simulink model "IdealGen_load_CtrlGen_wWT_abc_detailed_ver2"  (R2023b)
settings: Solver=VariableStepAuto  StartTime=0.0  StopTime=Tend  RelTol=1e-3
undefined symbols (not defined in the file): C_dc, c_drt, C_f, C_p_opt, f_nom, H_gen, H_vsm, H_WTR, I_dc_base, Ibase_hv, Ibase_lv, k_d_vsm, k_drt, k_p_p_vsm, k_p_q_vsm, K_pitch, Ki_cc, ki_q, Ki_vc, Kp_cc, Kp_vc, kpu, L_d, l_f, L_f, L_grid, L_mv, L_q, l_t_hvmv, l_t_mvlv, lambda_opt, Lbase1v, omega_nom, omega_WTR_min, omega_WTR_n, omega_WTR_sl, phase_shift_test_state, phase_shifts, pitch_max, pitch_min, Pitchanglevector, Pmax, Powercoefficient, psi_pm, R_a, r_f, R_grid, R_mv, r_t_hvmv, r_t_mvlv, R_WTR, rate_max, rate_min, rocof_slope, Rocof_test_state, Sbase1, Sbase_t1, T_base, T_pitch, T_servo ... (+15)
libraries: spsControlledVoltageSourceLib x6, slpidlib x6, spsPower3phInstantaneousLib x4, spsThreePhaseSeriesRLCBranchLib x4, spsThreePhaseVIMeasurementLib x3, spsRMSLib x3, spsabctodq0Lib x3, spsGroundLib x2, spsdq0toabcLib x2, spsCurrentMeasurementLib x2, spsSeriesRLCBranchLib x2, spsVoltageMeasurementLib x2
(part 2 of 2)

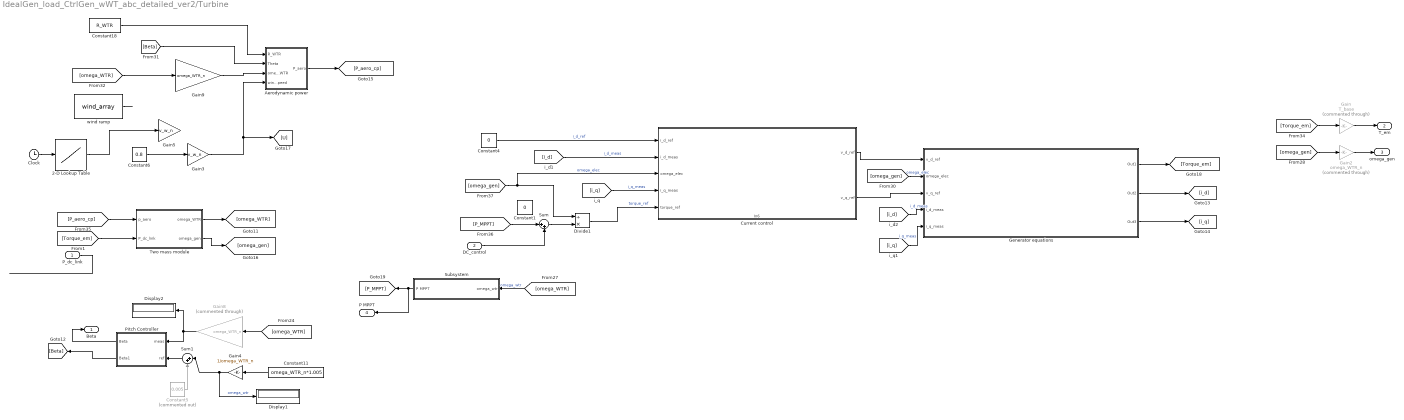
== system IdealGen_load_CtrlGen_wWT_abc_detailed_ver2/Turbine ==
  P_dc_link : Inport
  DC_control : Inport  Port=2
  2-D Lookup Table : Lookup_n-D  NumberOfTableDimensions=1  BreakpointsForDimension1=wind_array_step(1,:)  BreakpointsForDimension2=[1:3]  IndexSearchMethod=Linear search  Table=wind_array_step(2,:)  InterpMethod=Nearest  InternalRulePriority=Speed  RndMeth=Simplest
  Aerodynamic power : Subsystem
  Clock : Clock
  Constant1 : Constant  Value=0
  Constant11 : Constant  Value=omega_WTR_n*1.005
  Constant18 : Constant  Value=R_WTR
  Constant4 : Constant  Value=0
  Constant5 : Constant  Commented=on  Value=0.005
  Constant6 : Constant  Value=0.8
  Current control : Subsystem
      settings: PortSchema="{\"entries\":[{\"content\":{\"sides\":[{\"content\":{\"connectorIds\":[\"In1\",\"In2\",\"In3\",\"In4\",\"In5\"]},\"type\":\"ConnectorPlacement.EquallySpacedRectSide\",\"uuid\":\"f0c0ebaa-c967-4356-ac1b-c57f63a29779\"},{\"content\":{\"connectorIds\":[\"Out1\",\"Out2\"],\"side\":\"RIGHT\"},\"type\":\"ConnectorPlacement.EquallySpacedRectSide\",\"uuid\":\"1cdf54d9-8841-4054-96d8-98f023823611\"},{\"content\":{\"side\":\"TOP\"},\"type\":\"ConnectorPlacement.EquallySpacedRectSide\",\"uuid\":\"e5446ced-f102-4515-b1a2-d62d39d31328\"},{\"content\":{\"connectorIds\":[\"In6\"],\"side\":\"BOTTOM\"},\"type\":\"ConnectorPlacement.EquallySpacedRectSide\",\"uuid\":\"501a05db-372f-49fd-99c3-d79253c332da\"}]},\"type\":\"ConnectorPlacement.EquallySpacedConnector\",\"uuid\":\"99b5cc9b-ee78-4a5c-8cde-7a0c5c1e273f\"}],\"packageUris\":[\"http://schema.mathworks.com/mf0/Connector/R2020b\"],\"version\":\"1.0\"}"
  Display1 : Display
  Display2 : Display
  Divide1 : Product  Inputs=/*
  Gain : Gain  Commented=through  Gain=T_base
  Gain2 : Gain  Commented=through  Gain=omega_WTR_n
  Gain3 : Gain  Gain=v_w_n
  Gain4 : Gain  Gain=1/omega_WTR_n
  Gain5 : Gain  Gain=v_w_n
  Gain8 : Gain  Commented=through  Gain=omega_WTR_n
  Gain9 : Gain  Gain=omega_WTR_n
  Generator equations : Subsystem
  Pitch Controller : Subsystem
  Subsystem : Subsystem
  Sum : Sum  Inputs=|++
  Sum1 : Sum  Inputs=|++
  Two mass module : Subsystem
  wind ramp : FromWorkspace  VariableName=wind_array
  Beta : Outport
  T_em : Outport  Port=2
  omega_gen : Outport  Port=3
  P MPPT : Outport  Port=4
  wires:
  [omega_gen] -> Gain2/1
  [omega_WTR] -> Subsystem/1(omega_wtr)  "omega_wtr"
  [i_d] -> Current control/2(i_d_meas)  "i_d_meas"
  Generator equations/3(Out3) -> [i_q]
  [i_q] -> Generator equations/5(i_q_meas)  "i_q_meas"
  Pitch Controller/1(Beta) -> Beta/1
  [i_d] -> Generator equations/4(i_d_meas)  "i_d_meas"
  Constant18/1 -> Aerodynamic power/1(R_WTR)
  [omega_gen] -> Generator equations/2(omega_elec)  "omega_elec"
  Gain3/1 -> Aerodynamic power/4(wind speed), [U]
  [Torque_em] -> Two mass module/2(P_dc_link)
  Constant11/1 -> Gain4/1
  wind ramp/1 -> ?
  [P_aero_cp] -> Two mass module/1(p_aero)
  Constant4/1 -> Current control/1(i_d_ref)  "i_d_ref"
  Generator equations/1(Out1) -> [Torque_em]
  Constant5/1 -> Sum1/2
  Two mass module/1(omega_WTR) -> [omega_WTR]
  [P_MPPT] -> Sum/1
  Two mass module/2(omega_gen) -> [omega_gen]
  [omega_gen] -> Divide1/1, Current control/3(omega_elec)  "omega_elec"
  Sum1/1 -> Pitch Controller/2(ref)
  Gain4/1 -> Sum1/1, Display1/1  "omega_wtr"
  Constant6/1 -> Gain3/1
  [omega_WTR] -> Gain8/1
  Clock/1 -> 2-D Lookup Table/1
  Pitch Controller/2(Beta1) -> [Beta]
  [i_q] -> Current control/4(i_q_meas)  "i_q_meas"
  Aerodynamic power/1(P_aero) -> [P_aero_cp]
  Gain9/1 -> Aerodynamic power/3(omega_WTR)
  Gain8/1 -> Display2/1, Pitch Controller/1(meas)
  [Beta] -> Aerodynamic power/2(Theta)
  2-D Lookup Table/1 -> Gain5/1
  [Torque_em] -> Gain/1
  Subsystem/1(P MPPT) -> P MPPT/1, [P_MPPT]
  Divide1/1 -> Current control/5(torque_ref)  "torque_ref"
  Current control/1(v_d_ref) -> Generator equations/1(v_d_ref)
  Generator equations/2(Out2) -> [i_d]
  [omega_WTR] -> Gain9/1
  Current control/2(v_q_ref) -> Generator equations/3(v_q_ref)
  Gain/1 -> T_em/1
  Gain2/1 -> omega_gen/1
  Sum/1 -> Divide1/2
  P_dc_link/1 -> ?
  DC_control/1 -> Sum/2

== system IdealGen_load_CtrlGen_wWT_abc_detailed_ver2/Voltage control ==
  Qm : Inport
  Qref : Inport  Port=2
  Constant5 : Constant
  Gain8 : Gain  Gain=1/Sbase1
  Gain9 : Gain  Gain=k_p_q_vsm
  Scope : Scope  NumInputPorts=4
  Sum3 : Sum  Inputs=|-+
  Sum4 : Sum  Inputs=|++
  Transfer Fcn1 : TransferFcn  Numerator=[ki_q]  Denominator=[1 ki_q]
  Vref : Outport
  delta Q : Outport  Port=2
  wires:
  Constant5/1 -> Sum4/2
  Qm/1 -> Gain8/1
  Gain9/1 -> Scope/3, Sum4/1
  Transfer Fcn1/1 -> Scope/2, Gain9/1
  Sum3/1 -> Transfer Fcn1/1, Scope/1, delta Q/1  "delta Q"
  Sum4/1 -> Scope/4, Vref/1  "Vref"
  Qref/1 -> Sum3/2
  Gain8/1 -> Sum3/1

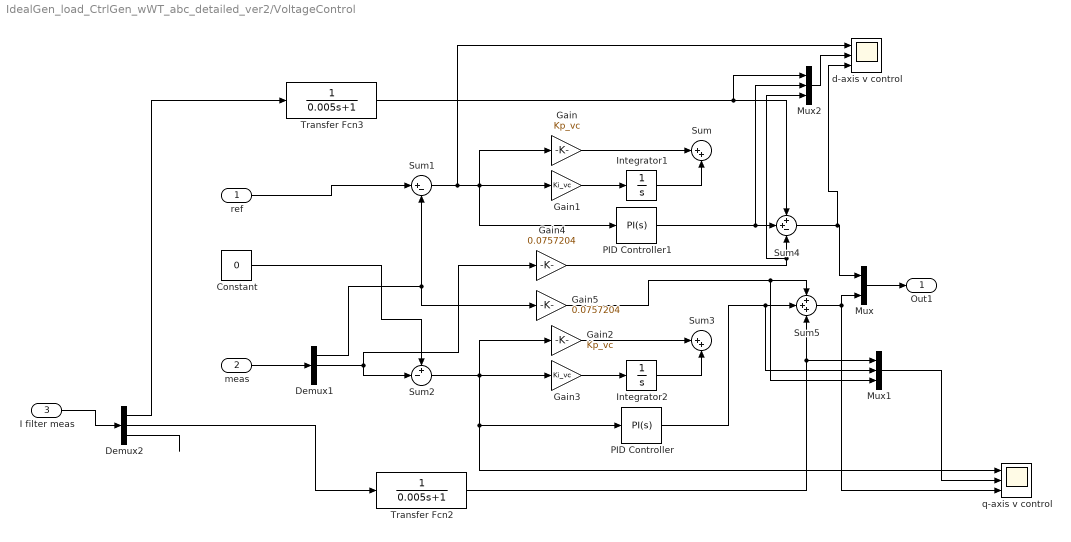
== system IdealGen_load_CtrlGen_wWT_abc_detailed_ver2/VoltageControl ==
  ref : Inport
  meas : Inport  Port=2
  I filter meas : Inport  Port=3
  Constant : Constant  Value=0
  Demux1 : Demux  Outputs=3
  Demux2 : Demux  Outputs=3
  Gain : Gain  Gain=Kp_vc
  Gain1 : Gain  Gain=Ki_vc
  Gain2 : Gain  Gain=Kp_vc
  Gain3 : Gain  Gain=Ki_vc
  Gain4 : Gain  Gain=0.0757204
  Gain5 : Gain  Gain=0.0757204
  Integrator1 : Integrator
  Integrator2 : Integrator
  Mux : Mux  Inputs=2
  Mux1 : Mux  Inputs=3
  Mux2 : Mux  Inputs=3
  PID Controller : slpidlib/PID Controller  Controller=PI  Form=Ideal  TimeDomain=Continuous-time  UseExternalTs=off  SampleTime=-1  IntegratorMethod=Forward Euler  FilterMethod=Forward Euler  ControllerParametersSource=internal  P=kpu  I=1/Tnu  UseKiTs=off  D=0  N=100  UseFilter=on  TunerSelectOption=Transfer Function Based (PID Tuner App)  InitialConditionSource=internal  InitialConditionForIntegrator=0  InitialConditionForFilter=0  DifferentiatorICPrevScaledInput=0  ExternalReset=none  TrackingMode=off  Kt=1  LimitOutput=off  SatLimitsSource=internal  UpperSaturationLimit=2  LowerSaturationLimit=-2  LinearizeAsGain=off  AntiWindupMode=none  Kb=1  LimitIntegrator=off  UpperIntegratorSaturationLimit=inf  LowerIntegratorSaturationLimit=-inf  POutMin=[]  POutMax=[]  IOutMin=[]  IOutMax=[]  DOutMin=[]  DOutMax=[]  NOutMin=[]  NOutMax=[]  SumOutMin=[]  SumOutMax=[]  SaturationOutMin=[]  SaturationOutMax=[]  PParamMin=[]  PParamMax=[]  IParamMin=[]  IParamMax=[]  DParamMin=[]  DParamMax=[]  NParamMin=[]  NParamMax=[]  KbParamMin=[]  KbParamMax=[]  KtParamMin=[]  KtParamMax=[]  KbOutMin=[]  KbOutMax=[]  KtOutMin=[]  KtOutMax=[]  IntegratorOutMin=[]  IntegratorOutMax=[]  FilterOutMin=[]  FilterOutMax=[]  SumI1OutMin=[]  SumI1OutMax=[]  SumI2OutMin=[]  SumI2OutMax=[]  SumI3OutMin=[]  SumI3OutMax=[]  SumI4OutMin=[]  SumI4OutMax=[]  SumDOutMin=[]  SumDOutMax=[]  DifferentiatorOutMin=[]  DifferentiatorOutMax=[]  FilterDiffOutCoefMin=[]  FilterDiffOutCoefMax=[]  ReciprocalOutMin=[]  ReciprocalOutMax=[]  SumDenOutMin=[]  SumDenOutMax=[]  SumNumOutMin=[]  SumNumOutMax=[]  DivideOutMin=[]  DivideOutMax=[]  UdiffTsProdOutMin=[]  UdiffTsProdOutMax=[]  NTsProdOutMin=[]  NTsProdOutMax=[]  UintegralTsProdOutMin=[]  UintegralTsProdOutMax=[]  UngainTsProdOutMin=[]  UngainTsProdOutMax=[]  ClampingZeroOutDataTypeStr=Inherit: Inherit via back propagation  ClampingZeroOutMin=[]  ClampingZeroOutMax=[]  FilterDenConstantOutDataTypeStr=Inherit: Inherit via back propagation  FilterDenConstantOutMin=[]  FilterDenConstantOutMax=[]  PCopyOutDataTypeStr=Inherit: Inherit via back propagation  PCopyOutMin=[]  PCopyOutMax=[]  NCopyOutDataTypeStr=Inherit: Inherit via back propagation  NCopyOutMin=[]  NCopyOutMax=[]  IntegratorContinuousStateAttributes=''  IntegratorStateMustResolveToSignalObject=off  IntegratorRTWStateStorageClass=Auto  FilterContinuousStateAttributes=''  FilterStateMustResolveToSignalObject=off  FilterRTWStateStorageClass=Auto  ParallelPVariant=Passthrough  IdealPVariant=InternalParameters  IVariant=InternalParameters  DVariant=Disabled  IntegratorVariant=Continuous  SatVariant=Disabled  AWVariant=Passthrough  PCopyVariant=Disabled  TRVariant=Disabled  FdbkBlocksVariant=Forward  IdealPFdbkVariant=Disabled  SatFdbkVariant=Disabled  DerivativeFilterVariant=Disabled  NVariant=Disabled  NCopyVariant=Disabled_SignalSpec  FilterICVariant=Disabled  IntegratorICVariant=InternalICs  ExternalResetVariant=Disabled  TRSumVariant=Passthrough  SumFdbkVariant=Disabled  SumVariant=Sum_PI  TsampFilterVariant=InternalTs  TsampNgainVariant=Passthrough  TsampIntegralVariant=Disabled_SignalSpec  ExternalSaturationOutDataTypeStr=Inherit: Same as second input
  PID Controller1 : slpidlib/PID Controller  Controller=PI  Form=Ideal  TimeDomain=Continuous-time  UseExternalTs=off  SampleTime=-1  IntegratorMethod=Forward Euler  FilterMethod=Forward Euler  ControllerParametersSource=internal  P=kpu  I=1/Tnu  UseKiTs=off  D=0  N=100  UseFilter=on  TunerSelectOption=Transfer Function Based (PID Tuner App)  InitialConditionSource=internal  InitialConditionForIntegrator=1  InitialConditionForFilter=0  DifferentiatorICPrevScaledInput=0  ExternalReset=none  TrackingMode=off  Kt=1  LimitOutput=off  SatLimitsSource=internal  UpperSaturationLimit=2  LowerSaturationLimit=-2  LinearizeAsGain=off  AntiWindupMode=none  Kb=1  LimitIntegrator=off  UpperIntegratorSaturationLimit=inf  LowerIntegratorSaturationLimit=-inf  POutMin=[]  POutMax=[]  IOutMin=[]  IOutMax=[]  DOutMin=[]  DOutMax=[]  NOutMin=[]  NOutMax=[]  SumOutMin=[]  SumOutMax=[]  SaturationOutMin=[]  SaturationOutMax=[]  PParamMin=[]  PParamMax=[]  IParamMin=[]  IParamMax=[]  DParamMin=[]  DParamMax=[]  NParamMin=[]  NParamMax=[]  KbParamMin=[]  KbParamMax=[]  KtParamMin=[]  KtParamMax=[]  KbOutMin=[]  KbOutMax=[]  KtOutMin=[]  KtOutMax=[]  IntegratorOutMin=[]  IntegratorOutMax=[]  FilterOutMin=[]  FilterOutMax=[]  SumI1OutMin=[]  SumI1OutMax=[]  SumI2OutMin=[]  SumI2OutMax=[]  SumI3OutMin=[]  SumI3OutMax=[]  SumI4OutMin=[]  SumI4OutMax=[]  SumDOutMin=[]  SumDOutMax=[]  DifferentiatorOutMin=[]  DifferentiatorOutMax=[]  FilterDiffOutCoefMin=[]  FilterDiffOutCoefMax=[]  ReciprocalOutMin=[]  ReciprocalOutMax=[]  SumDenOutMin=[]  SumDenOutMax=[]  SumNumOutMin=[]  SumNumOutMax=[]  DivideOutMin=[]  DivideOutMax=[]  UdiffTsProdOutMin=[]  UdiffTsProdOutMax=[]  NTsProdOutMin=[]  NTsProdOutMax=[]  UintegralTsProdOutMin=[]  UintegralTsProdOutMax=[]  UngainTsProdOutMin=[]  UngainTsProdOutMax=[]  ClampingZeroOutDataTypeStr=Inherit: Inherit via back propagation  ClampingZeroOutMin=[]  ClampingZeroOutMax=[]  FilterDenConstantOutDataTypeStr=Inherit: Inherit via back propagation  FilterDenConstantOutMin=[]  FilterDenConstantOutMax=[]  PCopyOutDataTypeStr=Inherit: Inherit via back propagation  PCopyOutMin=[]  PCopyOutMax=[]  NCopyOutDataTypeStr=Inherit: Inherit via back propagation  NCopyOutMin=[]  NCopyOutMax=[]  IntegratorContinuousStateAttributes=''  IntegratorStateMustResolveToSignalObject=off  IntegratorRTWStateStorageClass=Auto  FilterContinuousStateAttributes=''  FilterStateMustResolveToSignalObject=off  FilterRTWStateStorageClass=Auto  ParallelPVariant=Passthrough  IdealPVariant=InternalParameters  IVariant=InternalParameters  DVariant=Disabled  IntegratorVariant=Continuous  SatVariant=Disabled  AWVariant=Passthrough  PCopyVariant=Disabled  TRVariant=Disabled  FdbkBlocksVariant=Forward  IdealPFdbkVariant=Disabled  SatFdbkVariant=Disabled  DerivativeFilterVariant=Disabled  NVariant=Disabled  NCopyVariant=Disabled_SignalSpec  FilterICVariant=Disabled  IntegratorICVariant=InternalICs  ExternalResetVariant=Disabled  TRSumVariant=Passthrough  SumFdbkVariant=Disabled  SumVariant=Sum_PI  TsampFilterVariant=InternalTs  TsampNgainVariant=Passthrough  TsampIntegralVariant=Disabled_SignalSpec  ExternalSaturationOutDataTypeStr=Inherit: Same as second input
  Sum : Sum  Inputs=|++
  Sum1 : Sum  Inputs=|+-
  Sum2 : Sum  Inputs=+-|
  Sum3 : Sum  Inputs=|++
  Sum4 : Sum  Inputs=++-
  Sum5 : Sum  Inputs=+++
  Transfer Fcn2 : TransferFcn  Denominator=[0.005 1]
  Transfer Fcn3 : TransferFcn  Denominator=[0.005 1]
  d-axis v control : Scope  NumInputPorts=3
  q-axis v control : Scope  NumInputPorts=3
  Out1 : Outport
  wires:
  Demux2/1 -> Transfer Fcn3/1
  I filter meas/1 -> Demux2/1
  Sum5/1 -> Mux/2, q-axis v control/3
  Demux2/2 -> Transfer Fcn2/1
  Sum4/1 -> Mux/1, d-axis v control/3
  Sum2/1 -> PID Controller/1, q-axis v control/1, Gain3/1, Gain2/1
  Gain2/1 -> Sum3/1
  Integrator2/1 -> Sum3/2
  Gain3/1 -> Integrator2/1
  PID Controller/1 -> Mux1/2, Sum5/2
  ref/1 -> Sum1/1
  Constant/1 -> Sum2/1
  Demux1/2 -> Sum2/2, Gain4/1
  meas/1 -> Demux1/1
  Sum1/1 -> PID Controller1/1, Gain/1, Gain1/1, d-axis v control/1
  Gain1/1 -> Integrator1/1
  Integrator1/1 -> Sum/2
  Gain/1 -> Sum/1
  Mux/1 -> Out1/1
  Demux2/3 -> ?
  Gain4/1 -> Mux2/3, Sum4/3
  Gain5/1 -> Mux1/3, Sum5/1
  Demux1/1 -> Sum1/2, Gain5/1
  PID Controller1/1 -> Mux2/2, Sum4/2
  Transfer Fcn3/1 -> Mux2/1, Sum4/1
  Mux1/1 -> q-axis v control/2
  Mux2/1 -> d-axis v control/2
  Transfer Fcn2/1 -> Sum5/3, Mux1/1

== system IdealGen_load_CtrlGen_wWT_abc_detailed_ver2/WT power ==
  I_dc : Inport
  Controlled Current Source : spsControlledCurrentSourceLib/Controlled Current Source  Initialize=on  Source_Type=DC  Amplitude=0  Phase=0  Frequency=0  Measurements=None
  Current Measurement1 : spsCurrentMeasurementLib/Current Measurement  PhasorSimulation=off  OutputType=Complex  PSBequivalent=0
  Memory1 : Memory  InitialCondition=V_dc
  Product1 : Product  SaturateOnIntegerOverflow=on  OutDataTypeStr=Inherit: Same as first input
  Voltage Measurement1 : spsVoltageMeasurementLib/Voltage Measurement  PhasorSimulation=off  OutputType=Complex  PSBequivalent=0
  + : PMIOPort  Side=Right
  - : PMIOPort  Port=2  Side=Right
  Pwt : Outport
  V_dc : Outport  Port=2
  i_dc_meas : Outport  Port=3
  wires:
  Current Measurement1/1 -> i_dc_meas/1, Product1/1
  Product1/1 -> Pwt/1
  Voltage Measurement1/1 -> Memory1/1, Product1/2
  I_dc/1 -> Controlled Current Source/1
  Memory1/1 -> V_dc/1
  connections:
  Controlled Current Source/LConn1 -- Voltage Measurement1/LConn2 -- -/RConn1
  Voltage Measurement1/LConn1 -- Current Measurement1/RConn1 -- +/RConn1
  Controlled Current Source/RConn1 -- Current Measurement1/LConn1

== system IdealGen_load_CtrlGen_wWT_abc_detailed_ver2/constant DC Voltage ==
  DC Voltage Source2 : spsDCVoltageSourceLib/DC Voltage Source  Amplitude=V_dc/2  Measurements=None
  DC Voltage Source3 : spsDCVoltageSourceLib/DC Voltage Source  Amplitude=V_dc/2  Measurements=None
  + : PMIOPort  Side=Left
  - : PMIOPort  Port=2  Side=Right
  connections:
  DC Voltage Source2/LConn1 -- DC Voltage Source3/RConn1
  DC Voltage Source2/RConn1 -- +/RConn1
  DC Voltage Source3/LConn1 -- -/RConn1

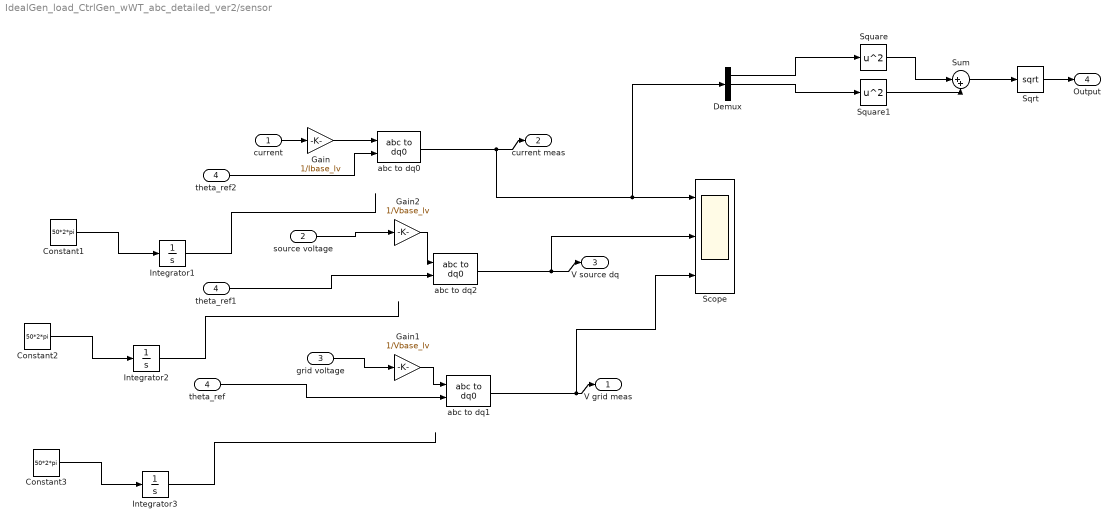
== system IdealGen_load_CtrlGen_wWT_abc_detailed_ver2/sensor ==
  current : Inport
  source voltage : Inport  Port=2
  grid voltage : Inport  Port=3
  theta_ref : Inport  Port=4
  Constant1 : Constant  Value=50*2*pi
  Constant2 : Constant  Value=50*2*pi
  Constant3 : Constant  Value=50*2*pi
  Demux : Demux  Outputs=3
  Gain : Gain  Gain=1/Ibase_lv
  Gain1 : Gain  Gain=1/Vbase_lv
  Gain2 : Gain  Gain=1/Vbase_lv
  Integrator1 : Integrator
  Integrator2 : Integrator
  Integrator3 : Integrator
  Scope : Scope  NumInputPorts=3
  Sqrt : Sqrt
  Square : Math  Operator=square
  Square1 : Math  Operator=square
  Sum : Sum  Inputs=|++
  abc to dq0 : spsabctodq0Lib/abc to dq0  Alignment=90 degrees behind phase A axis
  abc to dq1 : spsabctodq0Lib/abc to dq0  Alignment=90 degrees behind phase A axis
  abc to dq2 : spsabctodq0Lib/abc to dq0  Alignment=90 degrees behind phase A axis
  theta_ref1 : InportShadow  Port=4
  theta_ref2 : InportShadow  Port=4
  V grid meas : Outport
  current meas : Outport  Port=2
  V source dq : Outport  Port=3
  Output : Outport  Port=4
  wires:
  Gain/1 -> abc to dq0/1
  abc to dq0/1 -> Demux/1, Scope/1, current meas/1
  abc to dq1/1 -> Scope/3, V grid meas/1
  grid voltage/1 -> Gain1/1
  source voltage/1 -> Gain2/1
  abc to dq2/1 -> Scope/2, V source dq/1
  Integrator1/1 -> ?
  Constant1/1 -> Integrator1/1
  theta_ref/1 -> abc to dq1/2
  theta_ref1/1 -> abc to dq2/2
  theta_ref2/1 -> abc to dq0/2
  Constant2/1 -> Integrator2/1
  Integrator2/1 -> ?
  Integrator3/1 -> ?
  Constant3/1 -> Integrator3/1
  Gain2/1 -> abc to dq2/1
  current/1 -> Gain/1
  Gain1/1 -> abc to dq1/1
  Demux/1 -> Square/1
  Demux/2 -> Square1/1
  Square/1 -> Sum/1
  Square1/1 -> Sum/2
  Sum/1 -> Sqrt/1
  Sqrt/1 -> Output/1

== system IdealGen_load_CtrlGen_wWT_abc_detailed_ver2/DC-link voltage controller/DC init ==
  second : Inport
  init : Inport  Port=2
  Clock : Clock
  Switch : Switch  Criteria=u2 > Threshold  Threshold=10  SaturateOnIntegerOverflow=off  InputSameDT=off
  "   " : Outport
  wires:
  second/1 -> Switch/1
  init/1 -> Switch/3
  Clock/1 -> Switch/2
  Switch/1 -> "   "/1

== system IdealGen_load_CtrlGen_wWT_abc_detailed_ver2/Turbine/Aerodynamic power ==
  note: P = 0.5*rho*A*cp(lambda,beta)*U^3
  R_WTR : Inport
  Theta : Inport  Port=2
  omega_WTR : Inport  Port=3
  wind speed : Inport  Port=4
  2-D Lookup Table1 : Lookup_n-D  BreakpointsForDimension1=TSRvector  BreakpointsForDimension2=Pitchanglevector  Table=Powercoefficient  InternalRulePriority=Speed  RndMeth=Simplest
      settings: InputPortMap=u0,u1
  CP_calculator : MATLAB Function  TreatAsAtomicUnit=on
  CP_live : Scope  NumInputPorts=4
  Gain5 : Gain  Gain=1/v_w_n
  Gain7 : Gain  Gain=1/15e6
  MATLAB Function2 : MATLAB Function  TreatAsAtomicUnit=on
  Mux : Mux  Inputs=2
  P_aero_scope : Scope  NumInputPorts=3
  lambda_cal : MATLAB Function  TreatAsAtomicUnit=on
  P_aero : Outport
  wires:
  R_WTR/1 -> CP_calculator/2(R_WTR), MATLAB Function2/1(R_WTR)
  wind speed/1 -> Gain5/1, MATLAB Function2/3(U), CP_calculator/4(U), CP_live/3
  Theta/1 -> 2-D Lookup Table1/2, CP_live/1, CP_calculator/1(Theta)
  omega_WTR/1 -> CP_calculator/3(omega_WTR), CP_live/2
  MATLAB Function2/1(P_aero) -> Gain7/1
  CP_calculator/2(lambda) -> CP_live/4, 2-D Lookup Table1/1
  Gain7/1 -> P_aero_scope/1, P_aero/1  "p_aero [pu]"
  CP_calculator/1(cp) -> Mux/1
  Gain5/1 -> P_aero_scope/2  "Wind speed [pu]"
  2-D Lookup Table1/1 -> Mux/2, MATLAB Function2/2(cp)
  Mux/1 -> P_aero_scope/3  "Cp [pu]"

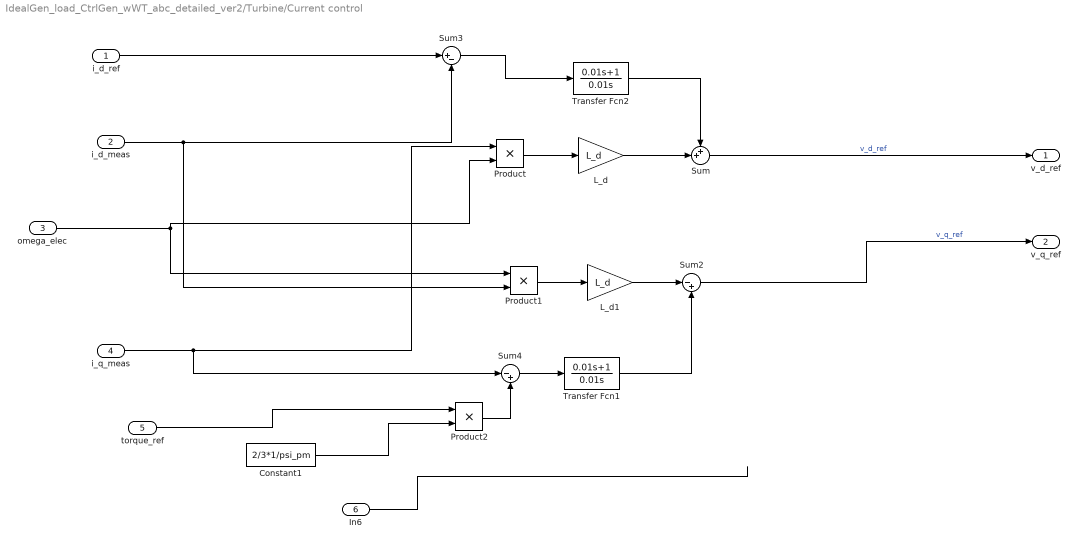
== system IdealGen_load_CtrlGen_wWT_abc_detailed_ver2/Turbine/Current control ==
  i_d_ref : Inport
  i_d_meas : Inport  Port=2
  omega_elec : Inport  Port=3
  i_q_meas : Inport  Port=4
  torque_ref : Inport  Port=5
  In6 : Inport  Port=6
  Constant1 : Constant  Value=2/3*1/psi_pm
  L_d : Gain  Gain=L_d
  L_d1 : Gain  Gain=L_d
  Product : Product
  Product1 : Product
  Product2 : Product
  Sum : Sum  Inputs=++|
  Sum2 : Sum  Inputs=|-+
  Sum3 : Sum  Inputs=|+-
  Sum4 : Sum  Inputs=|-+
  Transfer Fcn1 : TransferFcn  Numerator=[0.01 1]  Denominator=[0.01 0]
  Transfer Fcn2 : TransferFcn  Numerator=[0.01 1]  Denominator=[0.01 0]
  v_d_ref : Outport
  v_q_ref : Outport  Port=2
  wires:
  Sum3/1 -> Transfer Fcn2/1
  L_d1/1 -> Sum2/1
  Transfer Fcn2/1 -> Sum/1
  omega_elec/1 -> Product/2, Product1/1
  Constant1/1 -> Product2/2
  Sum4/1 -> Transfer Fcn1/1
  Product2/1 -> Sum4/2
  Product/1 -> L_d/1
  Sum/1 -> v_d_ref/1  "v_d_ref"
  Transfer Fcn1/1 -> Sum2/2
  i_d_meas/1 -> Product1/2, Sum3/2
  Product1/1 -> L_d1/1
  L_d/1 -> Sum/2
  i_q_meas/1 -> Sum4/1, Product/1
  i_d_ref/1 -> Sum3/1
  torque_ref/1 -> Product2/1
  Sum2/1 -> v_q_ref/1  "v_q_ref"
  In6/1 -> ?

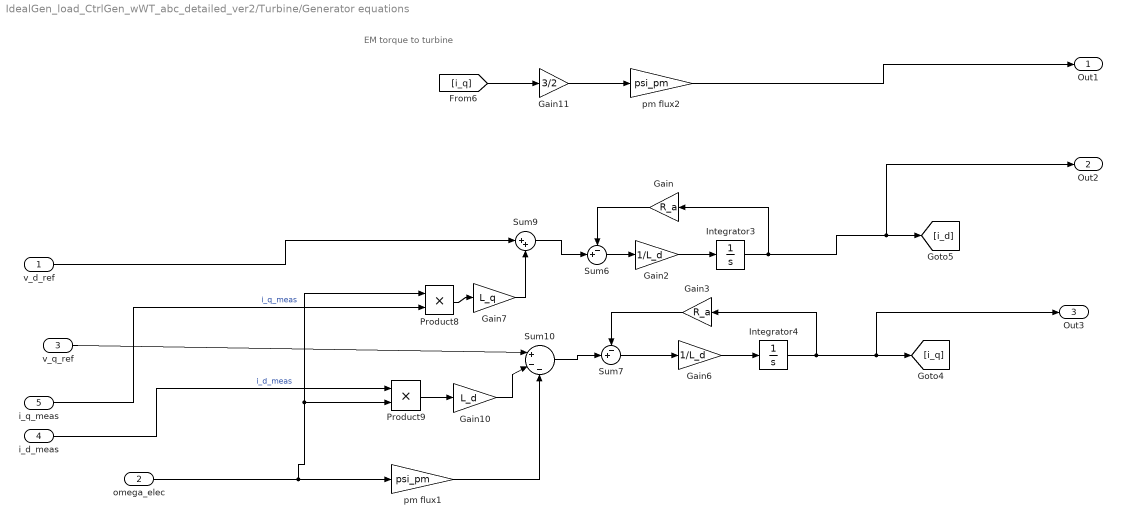
== system IdealGen_load_CtrlGen_wWT_abc_detailed_ver2/Turbine/Generator equations ==
  note: EM torque to turbine
  v_d_ref : Inport
  omega_elec : Inport  Port=2
  v_q_ref : Inport  Port=3
  i_d_meas : Inport  Port=4
  i_q_meas : Inport  Port=5
  Gain : Gain  Gain=R_a
  Gain10 : Gain  Gain=L_d
  Gain11 : Gain  Gain=3/2
  Gain2 : Gain  Gain=1/L_d
  Gain3 : Gain  Gain=R_a
  Gain6 : Gain  Gain=1/L_d
  Gain7 : Gain  Gain=L_q
  Integrator3 : Integrator
  Integrator4 : Integrator  InitialCondition=2.3e4
  Product8 : Product
  Product9 : Product
  Sum10 : Sum  Inputs=|+--
  Sum6 : Sum  Inputs=-+|
  Sum7 : Sum  Inputs=-+|
  Sum9 : Sum  Inputs=|++
  pm flux1 : Gain  Gain=psi_pm
  pm flux2 : Gain  Gain=psi_pm
  Out1 : Outport
  Out2 : Outport  Port=2
  Out3 : Outport  Port=3
  wires:
  Gain6/1 -> Integrator4/1
  Integrator4/1 -> Out3/1, [i_q], Gain3/1
  Sum10/1 -> Sum7/2
  v_d_ref/1 -> Sum9/1
  Product8/1 -> Gain7/1
  Sum7/1 -> Gain6/1
  Gain2/1 -> Integrator3/1
  pm flux1/1 -> Sum10/3
  Sum9/1 -> Sum6/2
  omega_elec/1 -> Product8/1, Product9/2, pm flux1/1
  [i_q] -> Gain11/1
  Gain3/1 -> Sum7/1
  Gain11/1 -> pm flux2/1
  Sum6/1 -> Gain2/1
  Gain10/1 -> Sum10/2
  Gain/1 -> Sum6/1
  Integrator3/1 -> Gain/1, Out2/1, [i_d]
  Product9/1 -> Gain10/1
  i_q_meas/1 -> Product8/2  "i_q_meas"
  i_d_meas/1 -> Product9/1  "i_d_meas"
  Gain7/1 -> Sum9/2
  v_q_ref/1 -> Sum10/1
  pm flux2/1 -> Out1/1

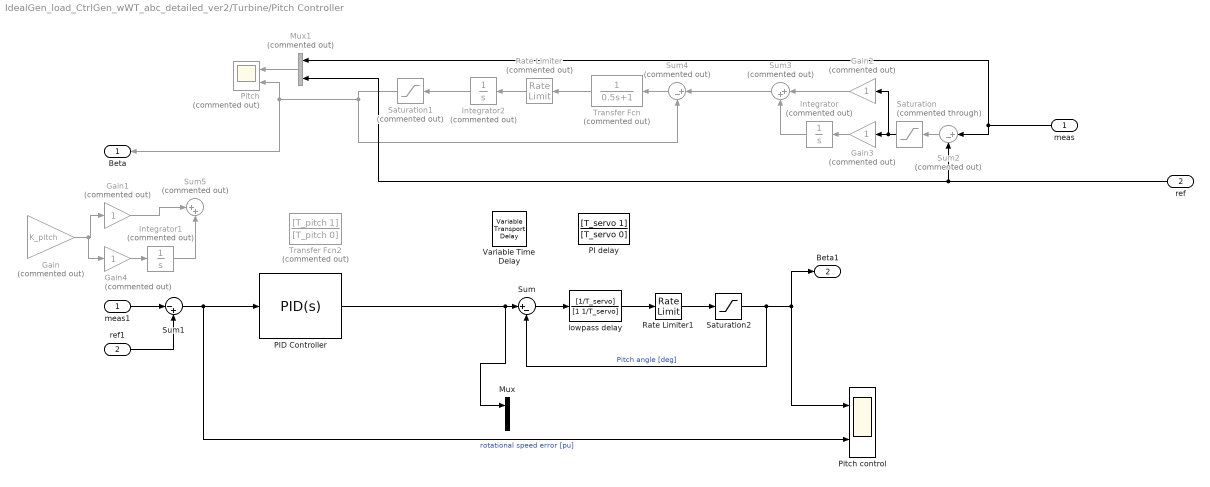
== system IdealGen_load_CtrlGen_wWT_abc_detailed_ver2/Turbine/Pitch Controller ==
  meas : Inport
  ref : Inport  Port=2
  Gain : Gain  Commented=on  Gain=K_pitch
  Gain{1..4} (4 alike) : Gain  Commented=on
  Integrator : Integrator  Commented=on
  Integrator1 : Integrator  Commented=on  LimitOutput=on  UpperSaturationLimit=pitch_max  LowerSaturationLimit=pitch_min
  Integrator2 : Integrator  Commented=on
  Mux : Mux  Inputs=2
  Mux1 : Mux  Commented=on  Inputs=2
  PI delay : TransferFcn  Numerator=[T_servo 1]  Denominator=[T_servo 0]
  PID Controller : slpidlib/PID Controller  Controller=PID  Form=Ideal  TimeDomain=Continuous-time  UseExternalTs=off  SampleTime=-1  IntegratorMethod=Forward Euler  FilterMethod=Forward Euler  ControllerParametersSource=internal  P=K_pitch  I=T_pitch  UseKiTs=on  D=0  N=100  UseFilter=on  TunerSelectOption=Transfer Function Based (PID Tuner App)  InitialConditionSource=internal  InitialConditionForIntegrator=0  InitialConditionForFilter=0  DifferentiatorICPrevScaledInput=0  ExternalReset=none  TrackingMode=off  Kt=1  LimitOutput=on  SatLimitsSource=internal  UpperSaturationLimit=pitch_max  LowerSaturationLimit=pitch_min  LinearizeAsGain=on  AntiWindupMode=clamping  Kb=1  LimitIntegrator=off  UpperIntegratorSaturationLimit=inf  LowerIntegratorSaturationLimit=-inf  POutMin=[]  POutMax=[]  IOutMin=[]  IOutMax=[]  DOutMin=[]  DOutMax=[]  NOutMin=[]  NOutMax=[]  SumOutMin=[]  SumOutMax=[]  SaturationOutMin=[]  SaturationOutMax=[]  PParamMin=[]  PParamMax=[]  IParamMin=[]  IParamMax=[]  DParamMin=[]  DParamMax=[]  NParamMin=[]  NParamMax=[]  KbParamMin=[]  KbParamMax=[]  KtParamMin=[]  KtParamMax=[]  KbOutMin=[]  KbOutMax=[]  KtOutMin=[]  KtOutMax=[]  IntegratorOutMin=[]  IntegratorOutMax=[]  FilterOutMin=[]  FilterOutMax=[]  SumI1OutMin=[]  SumI1OutMax=[]  SumI2OutMin=[]  SumI2OutMax=[]  SumI3OutMin=[]  SumI3OutMax=[]  SumI4OutMin=[]  SumI4OutMax=[]  SumDOutMin=[]  SumDOutMax=[]  DifferentiatorOutMin=[]  DifferentiatorOutMax=[]  FilterDiffOutCoefMin=[]  FilterDiffOutCoefMax=[]  ReciprocalOutMin=[]  ReciprocalOutMax=[]  SumDenOutMin=[]  SumDenOutMax=[]  SumNumOutMin=[]  SumNumOutMax=[]  DivideOutMin=[]  DivideOutMax=[]  UdiffTsProdOutMin=[]  UdiffTsProdOutMax=[]  NTsProdOutMin=[]  NTsProdOutMax=[]  UintegralTsProdOutMin=[]  UintegralTsProdOutMax=[]  UngainTsProdOutMin=[]  UngainTsProdOutMax=[]  ClampingZeroOutDataTypeStr=Inherit: Inherit via back propagation  ClampingZeroOutMin=[]  ClampingZeroOutMax=[]  FilterDenConstantOutDataTypeStr=Inherit: Inherit via back propagation  FilterDenConstantOutMin=[]  FilterDenConstantOutMax=[]  PCopyOutDataTypeStr=Inherit: Inherit via back propagation  PCopyOutMin=[]  PCopyOutMax=[]  NCopyOutDataTypeStr=Inherit: Inherit via back propagation  NCopyOutMin=[]  NCopyOutMax=[]  IntegratorContinuousStateAttributes=''  IntegratorStateMustResolveToSignalObject=off  IntegratorRTWStateStorageClass=Auto  FilterContinuousStateAttributes=''  FilterStateMustResolveToSignalObject=off  FilterRTWStateStorageClass=Auto  ParallelPVariant=Passthrough  IdealPVariant=InternalParameters  IVariant=InternalParameters  DVariant=InternalParameters  IntegratorVariant=Continuous  SatVariant=Enabled  AWVariant=ContClampingIdeal  PCopyVariant=InternalParamsIdeal  TRVariant=Disabled  FdbkBlocksVariant=Forward  IdealPFdbkVariant=Disabled  SatFdbkVariant=Disabled  DerivativeFilterVariant=ContFilter  NVariant=InternalParameters  NCopyVariant=Disabled  FilterICVariant=InternalICsFilter  IntegratorICVariant=InternalICs  ExternalResetVariant=Disabled  TRSumVariant=Passthrough  SumFdbkVariant=Disabled  SumVariant=Sum_PID  TsampFilterVariant=InternalTs  TsampNgainVariant=Passthrough  TsampIntegralVariant=Disabled_SignalSpec  ExternalSaturationOutDataTypeStr=Inherit: Same as second input
  Pitch : Scope  Commented=on  NumInputPorts=2
  Pitch control : Scope  NumInputPorts=2
  Rate Limiter : RateLimiter  Commented=on  RisingSlewLimit=5  FallingSlewLimit=-5  SampleTimeMode=inherited
  Rate Limiter1 : RateLimiter  RisingSlewLimit=rate_max  FallingSlewLimit=rate_min  SampleTimeMode=inherited
  Saturation : Saturate  Commented=through  UpperLimit=inf  LowerLimit=0
  Saturation1 : Saturate  Commented=on  UpperLimit=90  LowerLimit=0
  Saturation2 : Saturate  UpperLimit=pitch_max  LowerLimit=pitch_min
  Sum : Sum  Inputs=|+-
  Sum1 : Sum  Inputs=|-+
  Sum2 : Sum  Commented=on  Inputs=|+-
  Sum3 : Sum  Commented=on  Inputs=|++
  Sum4 : Sum  Commented=on  Inputs=|+-
  Sum5 : Sum  Commented=on  Inputs=|++
  Transfer Fcn : TransferFcn  Commented=on  Denominator=[0.5 1]
  Transfer Fcn2 : TransferFcn  Commented=on  Numerator=[T_pitch 1]  Denominator=[T_pitch 0]
  Variable Time Delay : VariableTransportDelay  MaximumDelay=T_servo
  lowpass delay : TransferFcn  Numerator=[1/T_servo]  Denominator=[1 1/T_servo]
  meas1 : InportShadow
  ref1 : InportShadow  Port=2
  Beta : Outport
  Beta1 : Outport  Port=2
  wires:
  Transfer Fcn/1 -> Rate Limiter/1
  meas/1 -> Sum2/1, Mux1/1
  Mux1/1 -> Pitch/1
  Sum2/1 -> Saturation/1
  Sum3/1 -> Sum4/1
  Saturation/1 -> Gain2/1, Gain3/1
  Saturation1/1 -> Beta/1, Pitch/2, Sum4/2
  Gain3/1 -> Integrator/1
  Gain2/1 -> Sum3/1
  Sum4/1 -> Transfer Fcn/1
  Rate Limiter/1 -> Integrator2/1
  Integrator/1 -> Sum3/2
  ref/1 -> Mux1/2, Sum2/2
  Integrator2/1 -> Saturation1/1
  Rate Limiter1/1 -> Saturation2/1
  Sum/1 -> lowpass delay/1
  lowpass delay/1 -> Rate Limiter1/1
  Saturation2/1 -> Beta1/1, Pitch control/1, Sum/2  "Pitch angle [deg]"
  meas1/1 -> Sum1/1
  ref1/1 -> Sum1/2
  PID Controller/1 -> Mux/1, Sum/1
  Sum1/1 -> PID Controller/1, Pitch control/2  "rotational speed error [pu]"
  Gain4/1 -> Integrator1/1
  Gain1/1 -> Sum5/1
  Integrator1/1 -> Sum5/2
  Gain/1 -> Gain4/1, Gain1/1

== system IdealGen_load_CtrlGen_wWT_abc_detailed_ver2/Turbine/Subsystem ==
  omega_wtr : Inport
  Constant12 : Constant  Value=R_WTR
  Constant13 : Constant  Value=lambda_opt
  Constant14 : Constant  Value=omega_WTR_n
  Constant15 : Constant  Value=omega_WTR_min
  Constant16 : Constant  Value=omega_WTR_sl
  Constant17 : Constant  Value=C_p_opt
  Gain10 : Gain  Commented=through  Gain=omega_WTR_n
  Gain11 : Gain  Commented=through  Gain=1/omega_WTR_n
  Gain12 : Gain  Gain=omega_WTR_n
  Gain6 : Gain  Gain=1/omega_WTR_n
  Gain7 : Gain  Gain=1/15e6
  MATLAB Function1 : MATLAB Function  TreatAsAtomicUnit=on
  MPPT : Scope  NumInputPorts=4
  P MPPT : Outport
  wires:
  Constant17/1 -> MATLAB Function1/6(cp_max)
  MATLAB Function1/2(b) -> MPPT/3
  Constant13/1 -> MATLAB Function1/4(lambda_opt)
  Gain6/1 -> MPPT/2  "omega_wtr"
  Gain7/1 -> P MPPT/1, MPPT/1
  Gain12/1 -> MATLAB Function1/7(omega_WTR), Gain6/1  "omega_wtr"
  Gain11/1 -> MATLAB Function1/3(omega_WTR_sl)  "omega_wtr"
  MATLAB Function1/1(P_MPPT) -> Gain7/1
  Constant15/1 -> MATLAB Function1/1(omega_WTR_min)
  Gain10/1 -> MATLAB Function1/2(omega_WTR_n)  "omega_wtr"
  Constant14/1 -> Gain10/1
  Constant16/1 -> Gain11/1
  Constant12/1 -> MATLAB Function1/5(R_WTR)
  MATLAB Function1/3(slope) -> MPPT/4
  omega_wtr/1 -> Gain12/1

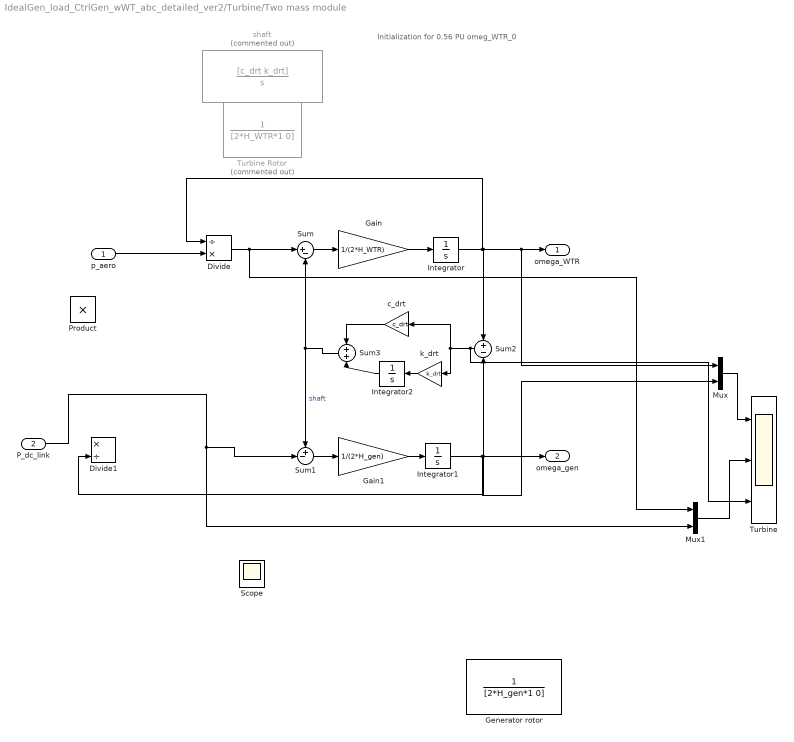
== system IdealGen_load_CtrlGen_wWT_abc_detailed_ver2/Turbine/Two mass module ==
  note: Initialization for 0.56 PU omeg_WTR_0
  p_aero : Inport
  P_dc_link : Inport  Port=2
  Divide : Product  Inputs=/*
  Divide1 : Product  Inputs=*/
  Gain : Gain  Gain=1/(2*H_WTR)
  Gain1 : Gain  Gain=1/(2*H_gen)
  Generator rotor : TransferFcn  Denominator=[2*H_gen*1 0]
  Integrator : Integrator  InitialCondition=omega_WTR_min/omega_WTR_n
  Integrator1 : Integrator  InitialCondition=omega_WTR_min/omega_WTR_n
  Integrator2 : Integrator
  Mux : Mux  Inputs=2
  Mux1 : Mux  Inputs=2
  Product : Product
  Scope : Scope  NumInputPorts=2
  Sum : Sum  Inputs=|+-
  Sum1 : Sum  Inputs=+-|
  Sum2 : Sum  Inputs=+|-
  Sum3 : Sum  Inputs=+|+
  Turbine : Scope  NumInputPorts=3
  Turbine Rotor : TransferFcn  Commented=on  Denominator=[2*H_WTR*1 0]
  c_drt : Gain  Gain=c_drt
  k_drt : Gain  Gain=k_drt
  shaft : TransferFcn  Commented=on  Numerator=[c_drt k_drt]  Denominator=[1 0]
  omega_WTR : Outport
  omega_gen : Outport  Port=2
  wires:
  Integrator1/1 -> Divide1/2, omega_gen/1, Sum2/2, Mux/2
  Sum3/1 -> Sum1/1, Sum/2  "shaft"
  Integrator/1 -> Divide/1, Mux/1, omega_WTR/1, Sum2/1
  Sum/1 -> Gain/1
  p_aero/1 -> Divide/2
  Gain/1 -> Integrator/1
  Gain1/1 -> Integrator1/1
  Sum1/1 -> Gain1/1
  Integrator2/1 -> Sum3/2
  c_drt/1 -> Sum3/1
  Sum2/1 -> Turbine/3, k_drt/1, c_drt/1
  k_drt/1 -> Integrator2/1
  Mux/1 -> Turbine/1
  Divide/1 -> Mux1/1, Sum/1
  Mux1/1 -> Turbine/2
  P_dc_link/1 -> Mux1/2, Sum1/2

== matlab function IdealGen_load_CtrlGen_wWT_abc_detailed_ver2/Turbine/Aerodynamic power/lambda_cal ==
  data: R_WTR input; omega_WTR input; U input; lambda output
function lambda  = fcn(R_WTR,omega_WTR,U) 
    
    lambda = omega_WTR*R_WTR/U;

== matlab function IdealGen_load_CtrlGen_wWT_abc_detailed_ver2/Turbine/Subsystem/MATLAB Function1 ==
  data: omega_WTR_min input; P_MPPT output; omega_WTR_n input; omega_WTR_sl input; lambda_opt input; R_WTR input; cp_max input; omega_WTR input; b output; slope output
function [P_MPPT,b,slope] = fcn(omega_WTR_min,omega_WTR_n,omega_WTR_sl,lambda_opt,R_WTR,cp_max,omega_WTR)

rho = 1.2225;
P_mppt_sl = 0.5*pi*rho*R_WTR^5*cp_max/lambda_opt^3*omega_WTR_sl^3; %
P_mppt_max = 0.5*pi*rho*R_WTR^5*cp_max/lambda_opt^3*omega_WTR_n^3;
slope = (P_mppt_max-P_mppt_sl)/(omega_WTR_n-omega_WTR_sl);
b = P_mppt_max-slope*omega_WTR_n;

if omega_WTR < omega_WTR_min*0.5
    y = 0;
elseif omega_WTR < omega_WTR_sl
    y = 0.5*pi*rho*R_WTR^5*cp_max/lambda_opt^3*omega_WTR^3;
elseif omega_WTR < omega_WTR_n % at 1.0236 pu the turbine reaches P = 15 MW 
    y  =slope*omega_WTR+b;
% 0.5*pi*rho*R_WTR^5*cp_zero_deg/lambda_not_opt^3*omega_WTR^3;
else
    y = 1.5e6;%0.5*pi*rho*R_WTR^5*cp_max/lambda_opt^3*(omega_WTR_n)^3;
    
end

P_MPPT = y ;

== matlab function IdealGen_load_CtrlGen_wWT_abc_detailed_ver2/Turbine/Aerodynamic power/MATLAB Function2 ==
  data: R_WTR input; cp input; P_aero output; U input
function P_aero = fcn(R_WTR,cp,U)

rho = 1.225;
P_aero = 0.5*pi*rho*R_WTR^2*cp*U^3;

== matlab function IdealGen_load_CtrlGen_wWT_abc_detailed_ver2/Turbine/Aerodynamic power/CP_calculator ==
  data: Theta input; R_WTR input; omega_WTR input; cp output; U input; lambda output
function  [cp, lambda] = fcn(Theta,R_WTR,omega_WTR,U) 
    
    lambda = omega_WTR*R_WTR/U;

    c = [0.645 116 0.4 5 21 0.00912 0.08 0.035 0.001];
    a = (-c(4)-c(3)*(2.5+Theta)+c(2)*1/(lambda+c(7)*(2.5+Theta))-c(8)/(lambda+(2.5+Theta)^3));
    exponent = c(5)*1/(lambda+c(7)*(2.5+Theta))-c(8)/(lambda+(2.5+Theta)^3);
    x = c(1)*(c(6)*lambda+a/exp(exponent))+c(9)*lambda;

cp = x;
